simulink model "linearizationPlant_cm"  (R2018b)
settings: Solver=FixedStepAuto  StartTime=0.0  StopTime=10.0  FixedStep=simulationTimeStep_s  MaxStep=simulationTimeStep_s  RelTol=1e-3
undefined symbols (not defined in the file): initialHeading_deg, initialPathPosition_none, initialSpeed_mPs, initialXPosition_m, initialYPosition_m
libraries: calculatePathSpeed x1, pathProjection_ul x1, stateEquations_ul x1
settings Model: Creator=mcobb  LastModifiedBy=mcobb
settings DebuggingCC: LibraryContextMissingDiagnostic=none
settings SFSimCC: SimUseLocalCustomCode=off
settings RTWCC: RTWUseLocalCustomCode=off

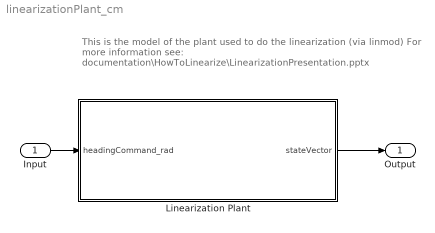
== system linearizationPlant_cm ==
  note: This is the model of the plant used to do the linearization (via linmod)
      | For more information see:
      | documentation\HowToLinearize\LinearizationPresentation.pptx
  Input : Inport
  Linearization Plant : Subsystem  AncestorBlock=linearizationPlant_cl/Linearization Plant  VariantControl=VSS_NONLINEAR_PLNT
  Output : Outport
  wires:
  Input/1 -> Linearization Plant/1(headingCommand_rad)
  Linearization Plant/1(stateVector) -> Output/1

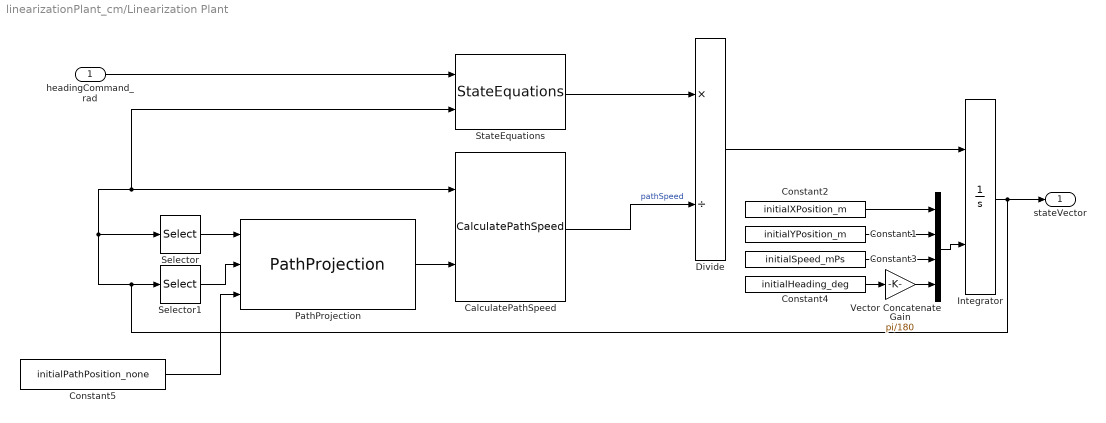
== system linearizationPlant_cm/Linearization Plant ==
  headingCommand_rad : Inport
  CalculatePathSpeed : calculatePathSpeed/CalculatePathSpeed  SystemSampleTime=-1
  Constant1 : Constant  Value=initialYPosition_m
  Constant2 : Constant  Value=initialXPosition_m
  Constant3 : Constant  Value=initialSpeed_mPs
  Constant4 : Constant  Value=initialHeading_deg
  Constant5 : Constant  Value=initialPathPosition_none
  Divide : Product  Inputs=*/
  Gain : Gain  Gain=pi/180
  Integrator : Integrator  InitialConditionSource=external
  PathProjection : pathProjection_ul/PathProjection  SystemSampleTime=-1
  Selector : Selector  InputPortWidth=4  IndexOptions=Index vector (dialog)  Indices=1  OutputSizes=1
  Selector1 : Selector  InputPortWidth=4  IndexOptions=Index vector (dialog)  Indices=2  OutputSizes=1
  StateEquations : stateEquations_ul/StateEquations  SystemSampleTime=-1
  Vector Concatenate : Concatenate  NumInputs=4
  stateVector : Outport
  wires:
  Constant5/1 -> PathProjection/3
  Gain/1 -> Vector Concatenate/4
  Constant4/1 -> Gain/1
  Vector Concatenate/1 -> Integrator/2
  Constant2/1 -> Vector Concatenate/1
  Constant1/1 -> Vector Concatenate/2
  Constant3/1 -> Vector Concatenate/3
  Divide/1 -> Integrator/1
  CalculatePathSpeed/1 -> Divide/2  "pathSpeed"
  StateEquations/1 -> Divide/1
  PathProjection/1 -> CalculatePathSpeed/2
  Selector1/1 -> PathProjection/2
  Integrator/1 -> stateVector/1, CalculatePathSpeed/1, StateEquations/2, Selector/1, Selector1/1
  Selector/1 -> PathProjection/1
  headingCommand_rad/1 -> StateEquations/1
